simulink model "suspension"  (R2020a)
settings: Solver=VariableStepAuto  StartTime=0.0  StopTime=100  RelTol=1e-3
model workspace (MAT data in the model file):
  b = Simulink.Parameter
  b.DataType = 'auto'
  b.Dimensions = [0 0]
  k1 = Simulink.Parameter
  k1.DataType = 'auto'
  k1.Dimensions = [0 0]
  k2 = Simulink.Parameter
  k2.DataType = 'auto'
  k2.Dimensions = [0 0]
  m1 = Simulink.Parameter
  m1.DataType = 'auto'
  m1.Dimensions = [0 0]
  m2 = Simulink.Parameter
  m2.DataType = 'auto'
  m2.Dimensions = [0 0]
settings Model: Creator=akhil singh  LastModifiedBy=akhil singh

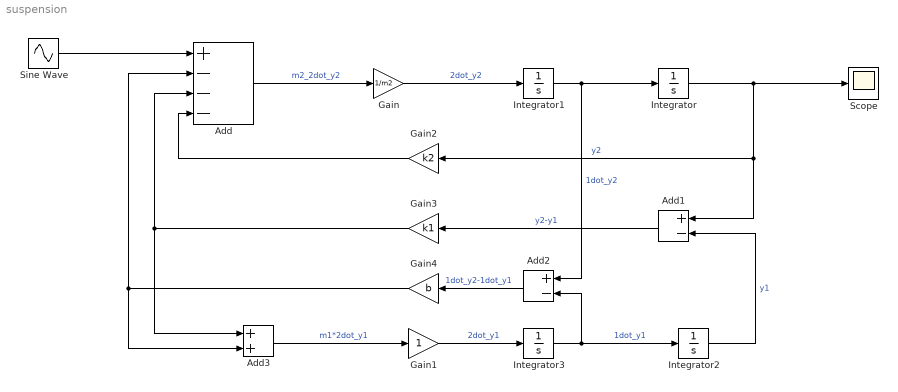
== system suspension ==
  Add : Sum  Inputs=+---
  Add1 : Sum  Inputs=+-
  Add2 : Sum  Inputs=+-
  Add3 : Sum
  Gain : Gain  Gain=1/m2
  Gain1 : Gain
  Gain2 : Gain  Gain=k2
  Gain3 : Gain  Gain=k1
  Gain4 : Gain  Gain=b
  Integrator : Integrator
  Integrator1 : Integrator  InitialCondition=1
  Integrator2 : Integrator
  Integrator3 : Integrator
  Scope : Scope
  Sine Wave : Sin  SampleTime=0
  wires:
  Sine Wave/1 -> Add/1
  Gain/1 -> Integrator1/1  "2dot_y2"
  Integrator1/1 -> Add2/1, Integrator/1  "1dot_y2"
  Add/1 -> Gain/1  "m2_2dot_y2"
  Integrator/1 -> Add1/1, Gain2/1, Scope/1  "y2"
  Gain2/1 -> Add/4
  Add1/1 -> Gain3/1  "y2-y1"
  Gain3/1 -> Add3/1, Add/3
  Gain1/1 -> Integrator3/1  "2dot_y1"
  Integrator2/1 -> Add1/2  "y1"
  Integrator3/1 -> Add2/2, Integrator2/1  "1dot_y1"
  Add2/1 -> Gain4/1  "1dot_y2-1dot_y1"
  Gain4/1 -> Add/2, Add3/2
  Add3/1 -> Gain1/1  "m1*2dot_y1"
